simulink model "simulink_lab3"  (R2018a)
settings: Solver=FixedStepDiscrete  StartTime=0.0  StopTime=12  FixedStep=1  RelTol=1e-3  EnableMultiTasking=on
libraries: dspsrcs4 x1
settings Model: Creator=cvillal3  LastModifiedBy=cvillal3

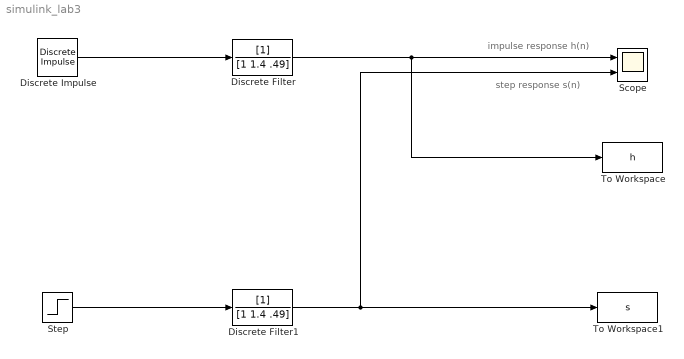
== system simulink_lab3 ==
  note: step response s(n)
  note: impulse response h(n)
  Discrete Impulse : dspsrcs4/Discrete  Impulse  Delay=0  SampleTime=1  FrameSample=1  OutputFrames=off  dataType=double  isSigned=on  wordLen=16  udDataType=sfix(16)  fracBitsMode=Best precision  numFracBits=15  OutDataTypeStr=double  LastOutDataTypeStr=double
  Discrete Filter : DiscreteFilter  Denominator=[1 1.4 .49]
  Discrete Filter1 : DiscreteFilter  Denominator=[1 1.4 .49]
  Scope : Scope  NumInputPorts=2
  Step : Step  Time=0  SampleTime=1
  To Workspace : ToWorkspace  VariableName=h  SaveFormat=Timeseries  SampleTime=-1
  To Workspace1 : ToWorkspace  VariableName=s  SaveFormat=Timeseries  SampleTime=-1
  wires:
  Discrete Impulse/1 -> Discrete Filter/1
  Step/1 -> Discrete Filter1/1
  Discrete Filter/1 -> To Workspace/1, Scope/1
  Discrete Filter1/1 -> Scope/2, To Workspace1/1
